simulink model "Q14"  (R2016b)
settings: Solver=VariableStepAuto  StartTime=0.0  StopTime=10.0  RelTol=1e-3
libraries: simulink x1
settings Model: Creator=AKSHAY JP PAWAR  LastModifiedBy=AKSHAY JP PAWAR
settings DataIOCC: ReturnWorkspaceOutputs=on
settings SFSimCC: SimUseLocalCustomCode=on
settings RTWCC: RTWUseLocalCustomCode=on

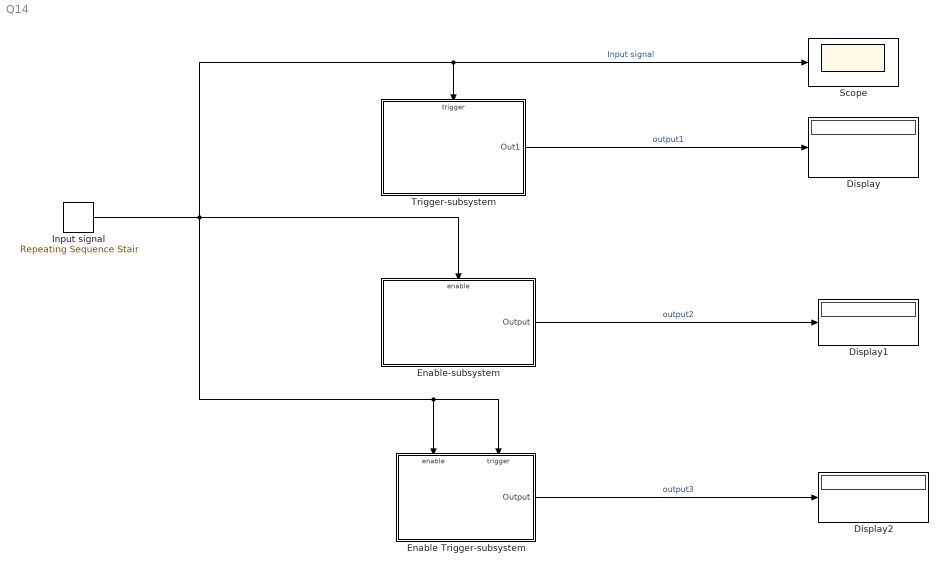
== system Q14 ==
  " Trigger-subsystem" : Subsystem
  Display : Display
  Display1 : Display
  Display2 : Display
  Enable Trigger-subsystem : Subsystem
  Enable-subsystem : Subsystem
  Input signal : simulink/Sources/Repeating Sequence Stair  OutValues=[0 1 1 0 0].'  tsamp=-1  OutMin=[]  OutMax=[]  OutDataTypeStr=double  OutputDataTypeScalingMode=double  OutDataType=fixdt(0,8)  ConRadixGroup=Best Precision: Vector-wise  OutScaling=2^-12
  Scope : Scope
  wires:
  Enable Trigger-subsystem/1(Output) -> Display2/1  "output3"
  Enable-subsystem/1(Output) -> Display1/1  "output2"
  " Trigger-subsystem"/1(Out1) -> Display/1  "output1"
  Input signal/1 -> Enable Trigger-subsystem/Trigger, Enable Trigger-subsystem/Enable, Enable-subsystem/Enable, Scope/1, " Trigger-subsystem"/Trigger  "Input signal"

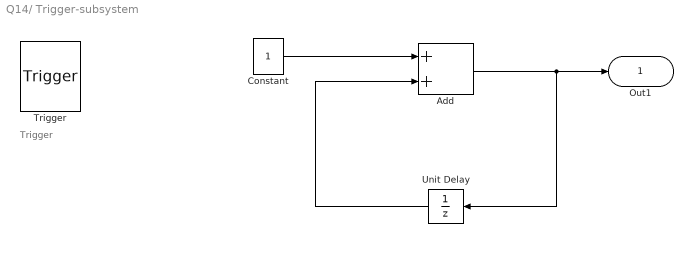
== system Q14/ Trigger-subsystem ==
  note: Trigger
  Trigger : TriggerPort  VariantControl=Variant  PortDimensions=1
  Add : Sum
  Constant : Constant
  Unit Delay : UnitDelay  SampleTime=-1  HasFrameUpgradeWarning=on
  Out1 : Outport
  wires:
  Constant/1 -> Add/1
  Add/1 -> Unit Delay/1, Out1/1
  Unit Delay/1 -> Add/2

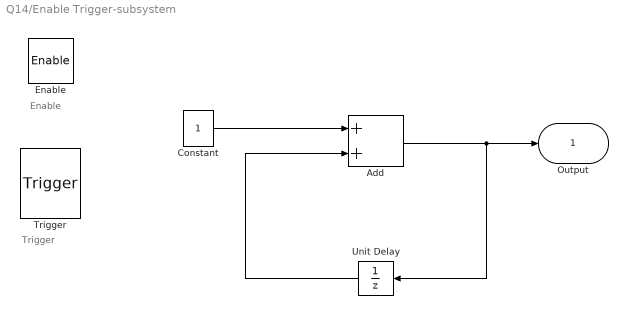
== system Q14/Enable Trigger-subsystem ==
  note: Trigger
  note: Enable
  Enable : EnablePort
  Trigger : TriggerPort  VariantControl=Variant  PortDimensions=1
  Add : Sum
  Constant : Constant
  Unit Delay : UnitDelay  SampleTime=-1  HasFrameUpgradeWarning=on
  Output : Outport
  wires:
  Constant/1 -> Add/1
  Add/1 -> Output/1, Unit Delay/1
  Unit Delay/1 -> Add/2

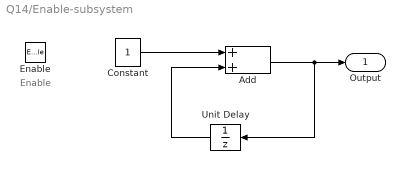
== system Q14/Enable-subsystem ==
  note: Enable
  Enable : EnablePort
  Add : Sum
  Constant : Constant
  Unit Delay : UnitDelay  SampleTime=-1  HasFrameUpgradeWarning=on
  Output : Outport
  wires:
  Constant/1 -> Add/1
  Add/1 -> Unit Delay/1, Output/1
  Unit Delay/1 -> Add/2
